simulink model "HWC_accel"  (R2018a)
settings: Solver=FixedStepAuto  StartTime=0.0  StopTime=stopTime  FixedStep=stepSize  RelTol=1e-3
values from neighbouring files (symbols this model uses):
  a = a_d    (= 6782.423)    [AA279D_hw4.m]    (also in AA279D_hw4_v2.m = 7500; SCHAUBprop.m = oe(1); TLE_Reader.m = (mu/n^2)^(1/3); keplerUniversal.m = 1./alpha(idx))
  mu = 398600    [AA279D_FINAL.m]    (also in AA279D_PSET1.m; AA279D_PSET2.m; AA279D_PSET2_a_change.m; AA279D_PSET3.m)
  rho_RTN_init = T_ECI2RTN*(r2_ECI_init-r_ECI_init)    [AA279D_PSET2.m]    (also in AA279D_PSET2_a_change.m; AA279D_PSET3.m; AA279D_PSET4.m; AA279D_hw4_v2.m)
  rhod_RTN_init = T_ECI2RTN*(v2_ECI_init-v_ECI_init)-     cross([0;0;thd0],rho_RTN_init)    [AA279D_PSET2.m]    (also in AA279D_PSET2_a_change.m; AA279D_PSET3.m; AA279D_PSET4.m; AA279D_hw4_v2.m)
settings Model: Creator=Christopher Covert  LastModifiedBy=Christopher Covert

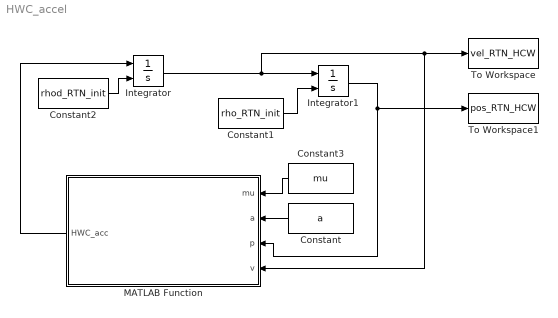
== system HWC_accel ==
  Constant : Constant  Value=a
  Constant1 : Constant  Value=rho_RTN_init
  Constant2 : Constant  Value=rhod_RTN_init
  Constant3 : Constant  Value=mu
  Integrator : Integrator  InitialConditionSource=external
  Integrator1 : Integrator  InitialConditionSource=external
  MATLAB Function : MATLAB Function  TreatAsAtomicUnit=on
  To Workspace : ToWorkspace  VariableName=vel_RTN_HCW  SampleTime=-1
  To Workspace1 : ToWorkspace  VariableName=pos_RTN_HCW  SampleTime=-1
  wires:
  Constant2/1 -> Integrator/2
  Integrator/1 -> Integrator1/1, MATLAB Function/4(v), To Workspace/1
  MATLAB Function/1(HWC_acc) -> Integrator/1
  Constant1/1 -> Integrator1/2
  Integrator1/1 -> To Workspace1/1, MATLAB Function/3(p)
  Constant3/1 -> MATLAB Function/1(mu)
  Constant/1 -> MATLAB Function/2(a)

== matlab function HWC_accel/MATLAB Function ==
  data: mu input; a input; HWC_acc output; p input; v input
function HWC_acc  = HWC_accel_prop(mu,a,p,v)

n = sqrt(mu/a^3);

xdd = 2*n*v(2)+3*n^2*p(1);
ydd = -2*n*v(1);
zdd = -n^2*p(3);

HWC_acc = [xdd,ydd,zdd];

end
